simulink model "PV_ES_System_mppt"  (R2024a)
settings: Solver=FixedStepDiscrete  StartTime=0.0  StopTime=4  FixedStep=1e-6  RelTol=1e-3
libraries: spsSeriesRLCBranchLib x5, spsDiodeLib x1, spsMosfetLib x1, spsPVArrayLib x1, SignalEditorBlockLib x1, spspowerguiLib x1
settings Model: Creator=ZE  LastModifiedBy=ZE

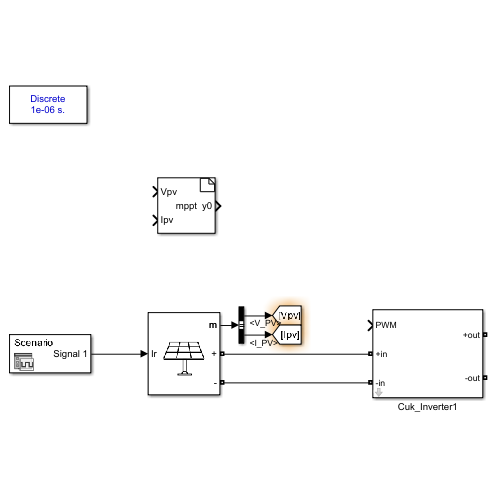
[thumbnail: Simulink's stored preview of the top-level diagram]
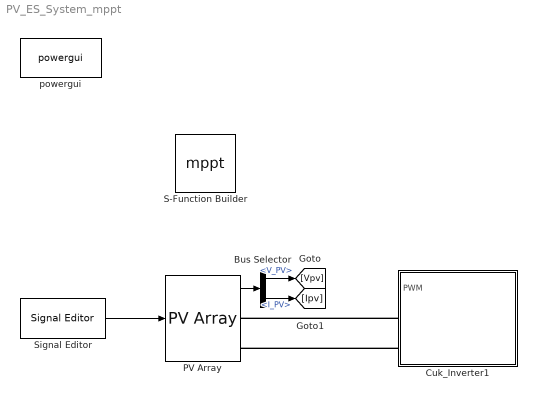
== system PV_ES_System_mppt ==
  Bus Selector : BusSelector  OutputSignals=V_PV,I_PV
  Cuk_Inverter1 : Subsystem  mask{Vin=30, Vout_Expect=40, Fsw=100e3, detaIL1=0.1, detaIL2=0.1, detaUC1=0.1, detaUC2=0.1}
      mask prompts: Fsw "Switch Frequency"; detaIL1 "电感纹波"; detaIL2 "电感纹波"; detaUC1 "电压纹波"; detaUC2 "电压纹波"
      mask DialogControl ParameterGroupVar Prompt: 参数
  PV Array : spsPVArrayLib/PV Array  Npar=10  Nser=1  PlotType=array @ 1000 W/m2 & specified temperatures  S_vec="[ 1000  500  100 ]"  Temp_C_vec="[ 45 25  ]"  ModuleName=A10Green Technology A10J-S72-175  PlotWhenSelected=off  Pm=175.0914  Ncell=72  Voc=43.99  Isc=5.17  Vm=36.63  Im=4.78  beta_Voc_pc=-0.3616  alpha_Isc_pc=0.041509  beta_Voc=-0.15907  alpha_Isc=0.002146  IL=5.178  I0=1.7842e-10  nI=0.98852  Rsh=249.6758  Rs=0.38412  RobustModel=on  RobustCellTemperature=25  BAL=on  Tc=1e-6  Tfilter=5e-5
  S-Function Builder : S-Function  FunctionName=mppt  SFunctionModules=mppt_wrapper.cpp  SFunctionDeploymentMode=off  EnableBusSupport=off  mask(S-Function Builder){}
      mask help: Simulink:masks:SFunctionBuilder_MD
      mask init:
      | val = [[.9  0.75 0.75 1 1 .9 .9 1]',[1 1 0.75 0.75 .9 .9 1 .9]'];try , sys = get_param(gcb,'SfunBuilderFcnName');if isempty(sys), sys = get_param(gcb,'FunctionName'); end,catch, sys = get_param(gcb,'FunctionName'); end
      settings: CopyFcn=set_param(gcbh,'LinkStatus','none')  OpenFcn=sfunctionwizard(gcbh)
      mask Display: plot(val(:,1),val(:,2)),disp(sys),port_label('input',1,'Vpv'),port_label('input',2,'Ipv'),port_label('output',1,'y0')
  Signal Editor : SignalEditorBlockLib/Signal Editor  FileName=C:\Users\ZE\Desktop\simulink_workspace\PV_ES_System(MPPT)\include\solar_Ir.mat  ActiveScenario=Scenario  ActiveSignal=Signal 1  IsBus=off  OutputBusObjectStr=Bus: BusObject  SampleTime=0  OutputAfterFinalValue=Holding final value  Unit=inherit  PreserveSignalName=on  ApplySigPropsToAllScenarios=on  ApplySigPropsToAllSignals=off
  powergui : spspowerguiLib/powergui  Priority=1  SimulationMode=Discrete  SampleTime=1e-6  frequency=60  Iterations=50  frequencyindice=0  Pbase=100e6  ErrMax=1e-4  UnitsV=kV  UnitsW=MW  buscounter=0  FunctionMessages=off  echomessages=off  EnableUseOfTLC=off  CurrentSourceSwitches=off  DisableSnubberDevices=off  DisableRonSwitches=off  DisableVfSwitches=off  DisplayEquations=off  AutomaticDiscreteSolvers=off  SolverType=Tustin/Backward Euler (TBE)  Interpol=off  ExternalGateDelay=off  methode=off  Ts=100  x0status=blocks  SPID=on  SwTol=0  HookPort=off  NonlinearTolerance=1e-4  nMaxIteration=100  ContinueOnMaxIteration=off  RestoreLinks=warning  ResistiveCurrentMeasurement=off  Frange=[0:2:500]  Ylog=off  Xlog=on  ShowGrid=off  save=off  variable=ZData  structure=0  ZoomFFT=off  StartTime=0.0  cycles=1  DisplayStyle=1  fundamental=60  FreqAxis=off  MaxFrequency=1000  frequencyindicesteady=1  RmsSteady=1  display=off
  wires:
  Signal Editor/1 -> PV Array/1
  PV Array/1 -> Bus Selector/1
  Bus Selector/1 -> [Vpv]  "<V_PV>"
  Bus Selector/2 -> [Ipv]  "<I_PV>"
  connections:
  Cuk_Inverter1/LConn1 -- PV Array/RConn1
  Cuk_Inverter1/LConn2 -- PV Array/RConn2

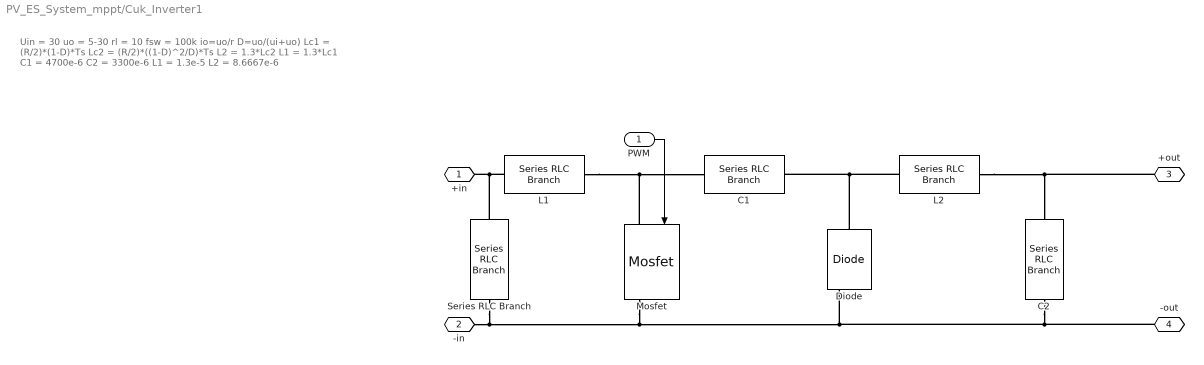
== system PV_ES_System_mppt/Cuk_Inverter1 ==
  note: Uin = 30
      | uo = 5-30
      | rl = 10
      | fsw = 100k
      | io=uo/r
      |
      | D=uo/(ui+uo)
      | Lc1 = (R/2)*(1-D)*Ts
      | Lc2 = (R/2)*((1-D)^2/D)*Ts
      | L2 = 1.3*Lc2
      | L1 = 1.3*Lc1
      | C1 = 4700e-6
      | C2 = 3300e-6
      |
      | L1 = 1.3e-5
      | L2 = 8.6667e-6
  PWM : Inport
  C1 : spsSeriesRLCBranchLib/Series RLC Branch  LConnTagsString=__new0  RConnTagsString=__new0  BranchType=C  Resistance=1  Inductance=1e-3  SetiL0=off  InitialCurrent=0  Capacitance=0.0047  Setx0=off  InitialVoltage=0  Measurements=None
  C2 : spsSeriesRLCBranchLib/Series RLC Branch  LConnTagsString=__new0  RConnTagsString=__new0  BranchType=C  Resistance=1  Inductance=1e-3  SetiL0=off  InitialCurrent=0  Capacitance=0.01  Setx0=off  InitialVoltage=0  Measurements=None
  Diode : spsDiodeLib/Diode  Ron=0.001  Lon=0  Vf=0.8  IC=0  UseSnubber=0  Rs=500  Cs=250e-9  Measurements=on
  L1 : spsSeriesRLCBranchLib/Series RLC Branch  LConnTagsString=__new0  RConnTagsString=__new0  BranchType=L  Resistance=1  Inductance=1e-3  SetiL0=off  InitialCurrent=0  Capacitance=1e-6  Setx0=off  InitialVoltage=0  Measurements=None
  L2 : spsSeriesRLCBranchLib/Series RLC Branch  LConnTagsString=__new0  RConnTagsString=__new0  BranchType=L  Resistance=1  Inductance=8.6667e-6  SetiL0=off  InitialCurrent=0  Capacitance=1e-6  Setx0=off  InitialVoltage=0  Measurements=None
  Mosfet : spsMosfetLib/Mosfet  Ron=0.1  Lon=0  Rd=0.01  Vfd=0  IC=0  Rs=1e5  Cs=inf  Measurements=on
  Series RLC Branch : spsSeriesRLCBranchLib/Series RLC Branch  LConnTagsString=__new0  RConnTagsString=__new0  BranchType=C  Resistance=1  Inductance=1e-3  SetiL0=off  InitialCurrent=0  Capacitance=1e-5  Setx0=off  InitialVoltage=0  Measurements=None
  +in : PMIOPort  Side=Left
  -in : PMIOPort  Port=2  Side=Left
  +out : PMIOPort  Port=3  Side=Right
  -out : PMIOPort  Port=4  Side=Right
  wires:
  PWM/1 -> Mosfet/1
  connections:
  L2/RConn1 -- +out/RConn1 -- C2/LConn1
  L2/LConn1 -- Diode/LConn1 -- C1/RConn1
  L1/LConn1 -- Series RLC Branch/LConn1 -- +in/RConn1
  L1/RConn1 -- Mosfet/LConn1 -- C1/LConn1
  Mosfet/RConn1 -- -in/RConn1 -- Series RLC Branch/RConn1 -- -out/RConn1 -- C2/RConn1 -- Diode/RConn1
